simulink library "mcadROM_lib"  (R2021b)
settings: Solver=VariableStepAuto  StartTime=0.0  StopTime=10.0  RelTol=1e-3
undefined symbols (not defined in the file): AdjMat, Banding_Loss_Mat, Friction_Loss_Mat, idx_TcoolantIn, idx_TcoolantOut, Iron_Loss_Rotor_Back_Iron_Mat, Iron_Loss_Rotor_Pole_Mat, Iron_Loss_Rotor_Tooth_Mat, Iron_Loss_Stator_Back_Iron_Mat, Iron_Loss_Stator_Tooth_Mat, Magnet_Loss_Mat, numStates, Rotor_Cage_Loss_Mat, ShaftTorqueVec, Sleeve_Loss_Mat, SpeedVec, StateSpaceND, Stator_Copper_Loss_AC_Mat, Stator_Copper_Loss_Mat, Stray_Load_Loss_Mat, Stray_Loss_Stator_Iron_Proportion, TnodesInit, Windage_Loss_Mat
libraries: cstblocks x2
settings Model: Creator=agonzale  LastModifiedBy=agonzale

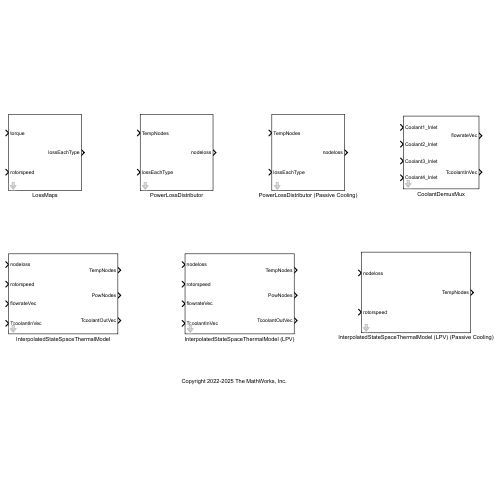
[thumbnail: Simulink's stored preview of the top-level diagram]
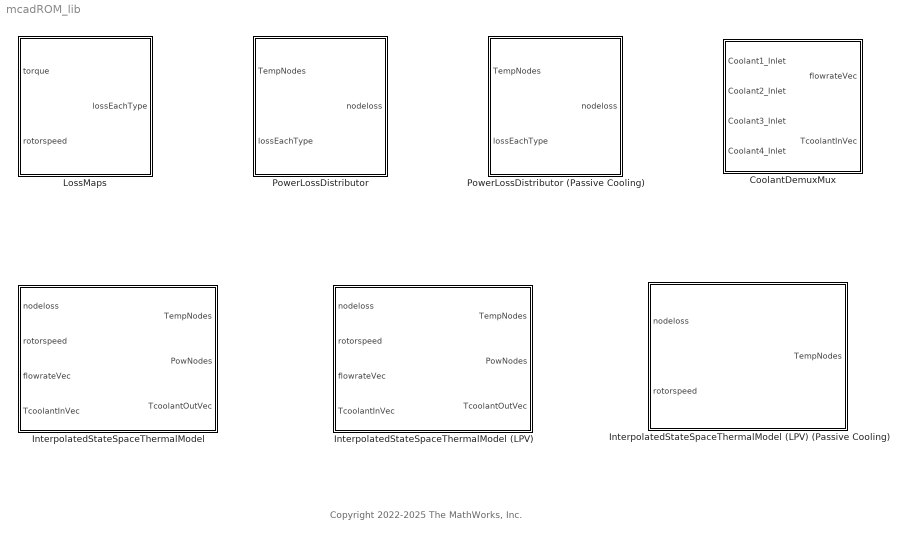
== system mcadROM_lib ==
  note: Copyright 2022-2025 The MathWorks, Inc.
  CoolantDemuxMux : Subsystem  mask{numCoolSys=4}
      mask prompts: numCoolSys "Number of cooling systems"
      mask init:
      | block_in2 = find_system(gcb, ...
      |     'LookUnderMasks', 'on', ...
      |     'FollowLinks', 'on', 'Name', 'Coolant2_Inlet');
      | 
      | block_in3 = find_system(gcb, ...
      |     'LookUnderMasks', 'on', ...
      |     'FollowLinks', 'on', 'Name', 'Coolant3_Inlet');
      | 
      | block_in4 = find_system(gcb, ...
      |     'LookUnderMasks', 'on', ...
      |     'FollowLinks', 'on', 'Name', 'Coolant4_Inlet');
      | 
      | ground2 = find_system(gcb, ...
      |     'LookUnderMasks', 'on', ...
      |     'FollowLinks', 'on', 'Name', 'Ground2');
      | 
      | ground3 = find_system(gcb, ...
      |     'LookUnderMasks', 'on', ...
      |     'FollowLinks', 'on', 'Name', 'Ground3');
      | 
      | ground4 = find_system(gcb, ...
      |     'LookUnderMasks', 'on', ...
      |     'FollowLinks', 'on', 'Name', 'Ground4');
      | 
      | Selector1 = [gcb, '/Selector1'];
      | Selector2 = [gcb, '/Selector2'];
      | 
      | switch numCoolSys
      |     case {1, '1'}
      | 	    set_param(Selector1, 'Indices', '1');
      |         set_param(Selector2, 'Indices', '1');
      |         if ~isempty(block_in2)
      |             delete_line(gcb, 'Coolant2_Inlet/1', 'Demux2/1');
      |             delete_block(block_in2);
      |         end
      |         if ~isempty(block_in3)
      |             delete_line(gcb, 'Coolant3_Inlet/1', 'Demux3/1');
      |             delete_block(block_in3);
      |         end
      |         if ~isempty(block_in4)
      |             delete_line(gcb, 'Coolant4_Inlet/1', 'Demux4/1');
      |             delete_block(block_in4);
      |         end
      |         if isempty(ground2)
      |             add_block('simulink/Sources/Ground', [gcb, '/Ground2']);
      |             add_line(gcb, 'Ground2/1', 'Demux2/1');
      |         end
      |         if isempty(ground3)
      |             add_block('simulink/Sources/Ground', [gcb, '/Ground3']);
      |             add_line(gcb, 'Ground3/1', 'Demux3/1');
      |         end
      |         if isempty(ground4)
      |             add_block('simulink/Sources/Ground', [gcb, '/Ground4']);
      |             add_line(gcb, 'Ground4/1', 'Demux4/1');
      |         end
      |     case {2, '2'}
      |         set_param(Selector1, 'Indices', '[1,2]');
      |         set_param(Selector2, 'Indices', '[1,2]');       
      |         if ~isempty(block_in3)
      |             delete_line(gcb, 'Coolant3_Inlet/1', 'Demux3/1');
      |             delete_block(block_in3);
      |         end
      |         if ~isempty(block_in4)
      |             delete_line(gcb, 'Coolant4_Inlet/1', 'Demux4/1');
      |             delete_block(block_in4);
      |         end 
      |         if ~isempty(ground2)
      |             delete_line(gcb, 'Ground2/1', 'Demux2/1');
      |             delete_block(ground2);
      |         end
      |         if isempty(block_in2)
      |             add_block('built-in/Inport', [gcb, '/Coolant2_Inlet']);
      |             add_line(gcb, 'Coolant2_Inlet/1', 'Demux2/1');
      |         end
      |         if isempty(ground3)
      |             add_block('simulink/Sources/Ground', [gcb, '/Ground3']);
      |             add_line(gcb, 'Ground3/1', 'Demux3/1');
      |         end
      |         if isempty(ground4)
      |             add_block('simulink/Sources/Ground', [gcb, '/Ground4']);
      |             add_line(gcb, 'Ground4/1', 'Demux4/1');
      |         end
      |     case {3, '3'}
      |         set_param(Selector1, 'Indices', '[1,2,3]');
      |         set_param(Selector2, 'Indices', '[1,2,3]');       
      |         if ~isempty(block_in4)          
      |             delete_line(gcb, 'Coolant4_Inlet/1', 'Demux4/1');
      |             delete_block(block_in4);
      |         end 
      |         if ~isempty(ground2)
      |             delete_line(gcb, 'Ground2/1', 'Demux2/1');
      |             delete_block(ground2);
      |         end
      |         if ~isempty(ground3)
      |             delete_line(gcb, 'Ground3/1', 'Demux3/1');
      |             delete_block(ground3);         
      |         end
      |         if isempty(block_in2)
      |             add_block('built-in/Inport', [gcb, '/Coolant2_Inlet']);
      |             add_line(gcb, 'Coolant2_Inlet/1', 'Demux2/1');
      |         end
      |         if isempty(block_in3)
      |             add_block('built-in/Inport', [gcb, '/Coolant3_Inlet']);
      |             add_line(gcb, 'Coolant3_Inlet/1', 'Demux3/1');
      |         end
      |         if isempty(ground4)
      |             add_block('simulink/Sources/Ground', [gcb, '/Ground4']);
      |             add_line(gcb, 'Ground4/1', 'Demux4/1');
      |         end
      |     case {4, '4'}
      |         set_param(Selector1, 'Indices', '[1,2,3,4]');
      |         set_param(Selector2, 'Indices', '[1,2,3,4]');
      |         if ~isempty(ground2)
      |             delete_line(gcb, 'Ground2/1', 'Demux2/1');
      |             delete_block(ground2);
      |         end
      |         if ~isempty(ground3)
      |             delete_line(gcb, 'Ground3/1', 'Demux3/1');
      |             delete_block(ground3);         
      |         end
      |         if ~isempty(ground4)
      |             delete_line(gcb, 'Ground4/1', 'Demux4/1');
      |             delete_block(ground4);
      |         end
      |         if isempty(block_in2)
      |             add_block('built-in/Inport', [gcb, '/Coolant2_Inlet']);
      |             add_line(gcb, 'Coolant2_Inlet/1', 'Demux2/1');
      |         end
      |         if isempty(block_in3)
      |             add_block('built-in/Inport', [gcb, '/Coolant3_Inlet']);
      |             add_line(gcb, 'Coolant3_Inlet/1', 'Demux3/1');
      |         end
      |         if isempty(block_in4)
      |             add_block('built-in/Inport', [gcb, '/Coolant4_Inlet']);
      |             add_line(gcb, 'Coolant4_Inlet/1', 'Demux4/1');
      |         end      
      | end
      mask TypeOptions numCoolSys: 1 | 2 | 3 | 4
  InterpolatedStateSpaceThermalModel : Subsystem  mask{BkptsStruct=struct('w', [1000,6000], 'fr1', [1,10], 'Tin1', [20,60]), AMatND=ones(3,2,2,50,50) % dummy value, BMatND=ones(3,2,2,50,50) % dummy value, ResMatND=ones(3,2,2,50,50) % dummy value, CoolAdjMat=zeros(50) % dummy value, CoolantArrayIdxs=[5 25] % dummy value, InletCoolantIdxs=[5] % dummy value, OutletCoolantIdxs=[25] % dummy value, TnodesInit=25*ones(50,1)}
      mask prompts: BkptsStruct "Speed and cooling inlet breakpoints (struct)"; AMatND "State-space A-matrix for each breakpoint"; BMatND "State-space B-matrix for each breakpoint"; ResMatND "Thermal resistance matrix for each breakpoint"; CoolAdjMat "Global cooling digraph adjacency matrix"; CoolantArrayIdxs "Coolant nodes indexes"; InletCoolantIdxs "Inlet node indexes for cooling systems"; OutletCoolantIdxs "Outlet node indexes for cooling systems"; TnodesInit "Initial node temperatures [degC]"
      mask init:
      | numStates = length(TnodesInit);
      | 
      | % numCoolSys = (length(Xcell)-1)/2;
      | % fieldnames = strings(1+2*numCoolSys,1);
      | % fieldNames(1) = "w";
      | % currentIdx = 2;
      | % for idxCool = 1:numCoolSys
      | %     fieldNames(currentIdx) = string(['fr',num2str(idxCool)]);
      | %     currentIdx = currentIdx+1;
      | % end
      | % for idxCool = 1:numCoolSys
      | %     fieldNames(currentIdx) = string(['Tin',num2str(idxCool)]);
      | %     currentIdx = currentIdx+1;
      | % end 
      | % 
      | % Xstruct = cell2struct(Xcell, fieldNames);
      | 
      | % numCoolSys = length(CoolingDataStruct.EnabledCoolingSystemNames);
      | % Xcell = cell(1+2*numCoolSys,1);
      | % Xcell{1} = RotorSpeedBkpts(:)';
      | % currentIdx = 2;
      | % for idxCool = 1:numCoolSys
      | %     Xcell{currentIdx} = CoolingDataStruct.FlowRateBkpts_lpm{idxCool}(:)';
      | %     currentIdx = currentIdx+1;
      | % end
      | % for idxCool = 1:numCoolSys
      | %     Xcell{currentIdx} = CoolingDataStruct.InletTempBkpts_degC{idxCool}(:)';
      | %     currentIdx = currentIdx+1;
      | % end
  InterpolatedStateSpaceThermalModel (LPV) : Subsystem  mask{StateSpaceND=StateSpaceND, CoolAdjMat=AdjMat, CoolantArrayIdxs=[idx_TcoolantIn, idx_TcoolantOut], InletCoolantIdxs=idx_TcoolantIn, OutletCoolantIdxs=idx_TcoolantOut, TnodesInit=TnodesInit}
      mask prompts: StateSpaceND "Array of state-space models"; CoolAdjMat "Global cooling digraph adjacency matrix"; CoolantArrayIdxs "Coolant nodes indexes"; InletCoolantIdxs "Inlet node indexes for cooling systems"; OutletCoolantIdxs "Outlet node indexes for cooling systems"; TnodesInit "Initial node temperatures [degC]"
      mask init:
      | numStates = length(TnodesInit);
  InterpolatedStateSpaceThermalModel (LPV) (Passive Cooling) : Subsystem  mask{StateSpaceND=StateSpaceND, TnodesInit=TnodesInit}
      mask prompts: StateSpaceND "Array of state-space models"; TnodesInit "Initial node temperatures [degC]"
      mask init:
      | numStates = length(TnodesInit);
  LossMaps : Subsystem  mask{ShaftTorqueVec=ShaftTorqueVec, SpeedVec=SpeedVec, Stator_Copper_Loss_Mat=Stator_Copper_Loss_Mat, Rotor_Cage_Loss_Mat=Rotor_Cage_Loss_Mat, Iron_Loss_Stator_Back_Iron_Mat=Iron_Loss_Stator_Back_Iron_Mat, Iron_Loss_Stator_Tooth_Mat=Iron_Loss_Stator_Tooth_Mat, Stray_Loss_Stator_Iron_Proportion=Stray_Loss_Stator_Iron_Proportion, Stray_Load_Loss_Mat=Stray_Load_Loss_Mat, Magnet_Loss_Mat=Magnet_Loss_Mat, Iron_Loss_Rotor_Pole_Mat=Iron_Loss_Rotor_Pole_Mat, Iron_Loss_Rotor_Back_Iron_Mat=Iron_Loss_Rotor_Back_Iron_Mat, Iron_Loss_Rotor_Tooth_Mat=Iron_Loss_Rotor_Tooth_Mat, Friction_Loss_Mat=Friction_Loss_Mat, Windage_Loss_Mat=Windage_Loss_Mat, Stator_Copper_Loss_AC_Mat=Stator_Copper_Loss_AC_Mat, Banding_Loss_Mat=Banding_Loss_Mat, Sleeve_Loss_Mat=Sleeve_Loss_Mat}
      mask prompts: ShaftTorqueVec "Shaft torque vector"; SpeedVec "Shaft speed vector"; Stator_Copper_Loss_Mat "Stator_Copper_Loss matrix"; Rotor_Cage_Loss_Mat "Rotor_Cage_Loss matrix"; Iron_Loss_Stator_Back_Iron_Mat "Iron_Loss_Stator_Back_Iron matrix"; Iron_Loss_Stator_Tooth_Mat "Iron_Loss_Stator_Tooth matrix"; Stray_Loss_Stator_Iron_Proportion "Stray Loss Stator Iron proportion"; Stray_Load_Loss_Mat "Stray_Load_Loss matrix"; Magnet_Loss_Mat "Magnet_Loss matrix"; Iron_Loss_Rotor_Pole_Mat "Iron_Loss_Rotor_Pole matrix"; Iron_Loss_Rotor_Back_Iron_Mat "Iron_Loss_Rotor_Back_Iron matrix"; Iron_Loss_Rotor_Tooth_Mat "Iron_Loss_Rotor_Tooth matrix"; Friction_Loss_Mat "Friction_Loss matrix"; Windage_Loss_Mat "Windage_Loss matrix"; Stator_Copper_Loss_AC_Mat "Stator_Copper_Loss_AC matrix"; Banding_Loss_Mat "Banding_Loss matrix"; Sleeve_Loss_Mat "Sleeve_Loss matrix"
  PowerLossDistributor : Subsystem  mask{TrefStator=20, StatorCopperTempCoefResistivity=1e-5, TrefRotor=20, RotorCopperTempCoefResistivity=1e-5, LossDistrForEachType=zeros(10,50);, CapMat=zeros(50);, CoolantArrayIdxs=[2,3,4]}
      mask prompts: TrefStator "Stator reference temperature [degC]"; StatorCopperTempCoefResistivity "Stator copper resistivity temperature coefficient"; TrefRotor "Rotor reference temperature [degC]"; RotorCopperTempCoefResistivity "Rotor copper resistivity temperature coefficient"; LossDistrForEachType "Node loss distribution for each loss type (array)"; CapMat "Capacitance matrix"; CoolantArrayIdxs "Coolant nodes indexes"
      mask init:
      | [numStates, ~] = size(CapMat);
  PowerLossDistributor (Passive Cooling) : Subsystem  mask{TrefStator=20, StatorCopperTempCoefResistivity=1e-5, TrefRotor=20, RotorCopperTempCoefResistivity=1e-5, LossDistrForEachType=zeros(10,50);, CapMat=zeros(50);}
      mask prompts: TrefStator "Stator reference temperature [degC]"; StatorCopperTempCoefResistivity "Stator copper resistivity temperature coefficient"; TrefRotor "Rotor reference temperature [degC]"; RotorCopperTempCoefResistivity "Rotor copper resistivity temperature coefficient"; LossDistrForEachType "Node loss distribution for each loss type (array)"; CapMat "Capacitance matrix"
      mask init:
      | [numStates, ~] = size(CapMat);

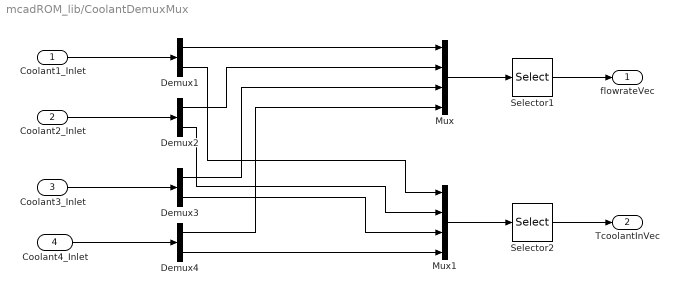
== system mcadROM_lib/CoolantDemuxMux ==
  Coolant1_Inlet : Inport
  Coolant2_Inlet : Inport  Port=2
  Coolant3_Inlet : Inport  Port=3
  Coolant4_Inlet : Inport  Port=4
  Demux{1..4} (4 alike) : Demux  Outputs=2
  Mux : Mux
  Mux1 : Mux
  Selector1 : Selector  InputPortWidth=4  IndexOptions=Index vector (dialog)  Indices=[1,2,3,4]  OutputSizes=1
  Selector2 : Selector  InputPortWidth=4  IndexOptions=Index vector (dialog)  Indices=[1,2,3,4]  OutputSizes=1
  flowrateVec : Outport
  TcoolantInVec : Outport  Port=2
  wires:
  Coolant1_Inlet/1 -> Demux1/1
  Demux1/1 -> Mux/1
  Demux2/1 -> Mux/2
  Demux3/1 -> Mux/3
  Demux4/1 -> Mux/4
  Demux1/2 -> Mux1/1
  Demux2/2 -> Mux1/2
  Demux3/2 -> Mux1/3
  Demux4/2 -> Mux1/4
  Mux/1 -> Selector1/1
  Selector1/1 -> flowrateVec/1
  Mux1/1 -> Selector2/1
  Selector2/1 -> TcoolantInVec/1
  Coolant2_Inlet/1 -> Demux2/1
  Coolant3_Inlet/1 -> Demux3/1
  Coolant4_Inlet/1 -> Demux4/1

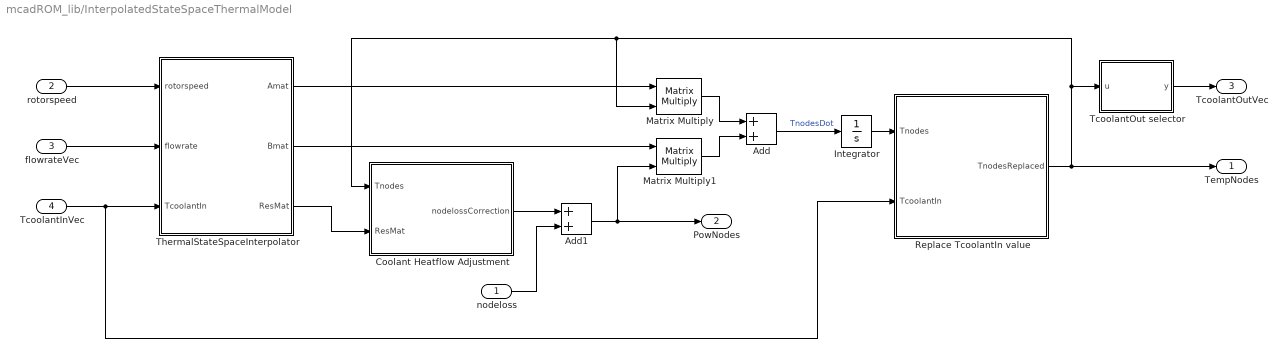
== system mcadROM_lib/InterpolatedStateSpaceThermalModel ==
  nodeloss : Inport
  rotorspeed : Inport  Port=2
  flowrateVec : Inport  Port=3
  TcoolantInVec : Inport  Port=4
  Add : Sum
  Add1 : Sum
  Coolant Heatflow Adjustment : MATLAB Function  TreatAsAtomicUnit=on
  Integrator : Integrator  InitialCondition=TnodesInit
  Matrix Multiply : Product  Multiplication=Matrix(*)
  Matrix Multiply1 : Product  Multiplication=Matrix(*)
  Replace TcoolantIn value : MATLAB Function  TreatAsAtomicUnit=on
  TcoolantOut selector : MATLAB Function  TreatAsAtomicUnit=on
  ThermalStateSpaceInterpolator : MATLAB Function  TreatAsAtomicUnit=on
  TempNodes : Outport
  PowNodes : Outport  Port=2
  TcoolantOutVec : Outport  Port=3
  wires:
  TcoolantOut selector/1(y) -> TcoolantOutVec/1
  Add1/1 -> PowNodes/1, Matrix Multiply1/2
  Matrix Multiply1/1 -> Add/2
  Integrator/1 -> Replace TcoolantIn value/1(Tnodes)
  Add/1 -> Integrator/1  "TnodesDot"
  Coolant Heatflow Adjustment/1(nodelossCorrection) -> Add1/1
  Matrix Multiply/1 -> Add/1
  Replace TcoolantIn value/1(TnodesReplaced) -> TempNodes/1, TcoolantOut selector/1(u), Matrix Multiply/2, Coolant Heatflow Adjustment/1(Tnodes)
  nodeloss/1 -> Add1/2
  TcoolantInVec/1 -> ThermalStateSpaceInterpolator/3(TcoolantIn), Replace TcoolantIn value/2(TcoolantIn)
  rotorspeed/1 -> ThermalStateSpaceInterpolator/1(rotorspeed)
  flowrateVec/1 -> ThermalStateSpaceInterpolator/2(flowrate)
  ThermalStateSpaceInterpolator/1(Amat) -> Matrix Multiply/1
  ThermalStateSpaceInterpolator/2(Bmat) -> Matrix Multiply1/1
  ThermalStateSpaceInterpolator/3(ResMat) -> Coolant Heatflow Adjustment/2(ResMat)

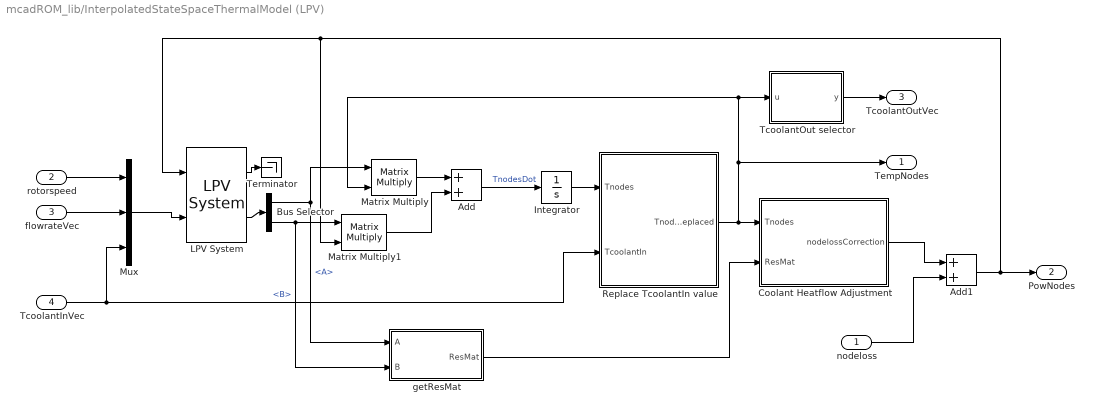
== system mcadROM_lib/InterpolatedStateSpaceThermalModel (LPV) ==
  nodeloss : Inport
  rotorspeed : Inport  Port=2
  flowrateVec : Inport  Port=3
  TcoolantInVec : Inport  Port=4
  Add : Sum
  Add1 : Sum
  Bus Selector : BusSelector  OutputSignals=A,B
  Coolant Heatflow Adjustment : MATLAB Function  TreatAsAtomicUnit=on
  Integrator : Integrator  InitialCondition=TnodesInit
  LPV System : cstblocks/Linear Parameter Varying/LPV System  sys=StateSpaceND  x0=TnodesInit  uOffset=0  yOffset=0  xOffset=0  opEquilOption=on  dxOffset=0  sysFixedOption=Use the first model in state-space array  sysFixed=[]  AFixed=false  BFixed=false  CFixed=false  DFixed=false  uDelayFixed=false  yDelayFixed=false  iDelayFixed=false  IMethod=Linear  EMethod=Clip  IndexSearch=Binary search  IndexBegin=on  OutputX=off  OutputXdot=off  OutputLTI=on  OutputOP=off  DataType=double  SimMode=Interpreted execution  InitBufferSize=1024  FixedBuffer=off
      settings: SourceProductBaseCode=CT
  Matrix Multiply : Product  Multiplication=Matrix(*)
  Matrix Multiply1 : Product  Multiplication=Matrix(*)
  Mux : Mux  Inputs=3
  Replace TcoolantIn value : MATLAB Function  TreatAsAtomicUnit=on
  TcoolantOut selector : MATLAB Function  TreatAsAtomicUnit=on
  Terminator : Terminator
  getResMat : MATLAB Function  TreatAsAtomicUnit=on
  TempNodes : Outport
  PowNodes : Outport  Port=2
  TcoolantOutVec : Outport  Port=3
  wires:
  Bus Selector/1 -> getResMat/1(A), Matrix Multiply/1  "<A>"
  LPV System/2 -> Bus Selector/1
  Integrator/1 -> Replace TcoolantIn value/1(Tnodes)
  Matrix Multiply1/1 -> Add/2
  Replace TcoolantIn value/1(TnodesReplaced) -> TempNodes/1, Matrix Multiply/2, TcoolantOut selector/1(u), Coolant Heatflow Adjustment/1(Tnodes)
  Matrix Multiply/1 -> Add/1
  Add/1 -> Integrator/1  "TnodesDot"
  Add1/1 -> PowNodes/1, LPV System/1, Matrix Multiply1/2
  Bus Selector/2 -> getResMat/2(B), Matrix Multiply1/1  "<B>"
  Coolant Heatflow Adjustment/1(nodelossCorrection) -> Add1/1
  getResMat/1(ResMat) -> Coolant Heatflow Adjustment/2(ResMat)
  Mux/1 -> LPV System/2
  TcoolantInVec/1 -> Replace TcoolantIn value/2(TcoolantIn), Mux/3
  nodeloss/1 -> Add1/2
  flowrateVec/1 -> Mux/2
  rotorspeed/1 -> Mux/1
  TcoolantOut selector/1(y) -> TcoolantOutVec/1
  LPV System/1 -> Terminator/1

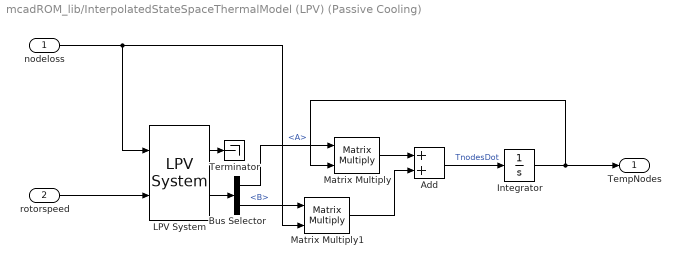
== system mcadROM_lib/InterpolatedStateSpaceThermalModel (LPV) (Passive Cooling) ==
  nodeloss : Inport
  rotorspeed : Inport  Port=2
  Add : Sum
  Bus Selector : BusSelector  OutputSignals=A,B
  Integrator : Integrator  InitialCondition=TnodesInit
  LPV System : cstblocks/Linear Parameter Varying/LPV System  sys=StateSpaceND  x0=TnodesInit  uOffset=0  yOffset=0  xOffset=0  opEquilOption=on  dxOffset=0  sysFixedOption=Use the first model in state-space array  sysFixed=[]  AFixed=false  BFixed=false  CFixed=false  DFixed=false  uDelayFixed=false  yDelayFixed=false  iDelayFixed=false  IMethod=Linear  EMethod=Clip  IndexSearch=Binary search  IndexBegin=on  OutputX=off  OutputXdot=off  OutputLTI=on  OutputOP=off  DataType=double  SimMode=Interpreted execution  InitBufferSize=1024  FixedBuffer=off
      settings: SourceProductBaseCode=CT
  Matrix Multiply : Product  Multiplication=Matrix(*)
  Matrix Multiply1 : Product  Multiplication=Matrix(*)
  Terminator : Terminator
  TempNodes : Outport
  wires:
  Bus Selector/1 -> Matrix Multiply/1  "<A>"
  LPV System/2 -> Bus Selector/1
  Matrix Multiply1/1 -> Add/2
  Integrator/1 -> Matrix Multiply/2, TempNodes/1
  Matrix Multiply/1 -> Add/1
  Add/1 -> Integrator/1  "TnodesDot"
  Bus Selector/2 -> Matrix Multiply1/1  "<B>"
  rotorspeed/1 -> LPV System/2
  LPV System/1 -> Terminator/1
  nodeloss/1 -> Matrix Multiply1/2, LPV System/1

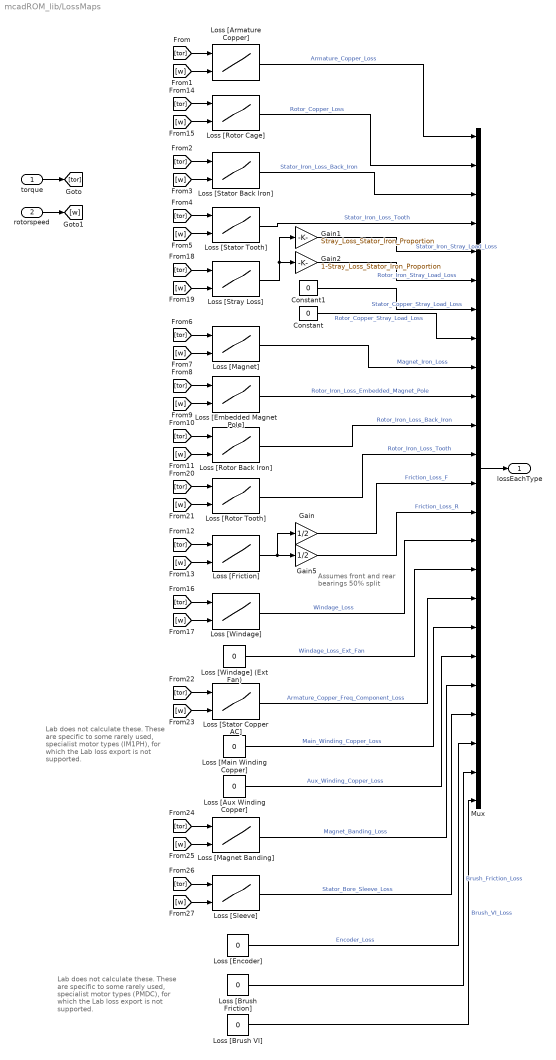
== system mcadROM_lib/LossMaps ==
  note: Lab does not calculate these.
      | These are specific to some rarely used, specialist  motor types (IM1PH), for which the Lab loss export is not supported.
  note: Assumes front and rear bearings 50% split
  note: Lab does not calculate these.
      | These are specific to some rarely used, specialist  motor types (PMDC), for which the Lab loss export is not supported.
  torque : Inport
  rotorspeed : Inport  Port=2
  Constant : Constant  Value=0
  Constant1 : Constant  Value=0
  Gain : Gain  Gain=1/2
  Gain1 : Gain  Gain=Stray_Loss_Stator_Iron_Proportion
  Gain2 : Gain  Gain=1-Stray_Loss_Stator_Iron_Proportion
  Gain5 : Gain  Gain=1/2
  Loss [Armature Copper] : Lookup_n-D  BreakpointsForDimension1=ShaftTorqueVec  BreakpointsForDimension2=SpeedVec  Table=Stator_Copper_Loss_Mat  ExtrapMethod=Clip  UseLastTableValue=on  InternalRulePriority=Speed  RndMeth=Simplest  InputSameDT=on
      settings: InputPortMap=u0,u1
  Loss [Aux Winding Copper] : Constant  Value=0
  Loss [Brush Friction] : Constant  Value=0
  Loss [Brush VI] : Constant  Value=0
  Loss [Embedded Magnet Pole] : Lookup_n-D  BreakpointsForDimension1=ShaftTorqueVec  BreakpointsForDimension2=SpeedVec  Table=Iron_Loss_Rotor_Pole_Mat  ExtrapMethod=Clip  UseLastTableValue=on  InternalRulePriority=Speed  RndMeth=Simplest  InputSameDT=on
      settings: InputPortMap=u0,u1
  Loss [Encoder] : Constant  Value=0
  Loss [Friction] : Lookup_n-D  BreakpointsForDimension1=ShaftTorqueVec  BreakpointsForDimension2=SpeedVec  Table=Friction_Loss_Mat  ExtrapMethod=Clip  UseLastTableValue=on  InternalRulePriority=Speed  RndMeth=Simplest  InputSameDT=on
      settings: InputPortMap=u0,u1
  Loss [Magnet Banding] : Lookup_n-D  BreakpointsForDimension1=ShaftTorqueVec  BreakpointsForDimension2=SpeedVec  Table=Banding_Loss_Mat  ExtrapMethod=Clip  UseLastTableValue=on  InternalRulePriority=Speed  RndMeth=Simplest  InputSameDT=on
      settings: InputPortMap=u0,u1
  Loss [Magnet] : Lookup_n-D  BreakpointsForDimension1=ShaftTorqueVec  BreakpointsForDimension2=SpeedVec  Table=Magnet_Loss_Mat  ExtrapMethod=Clip  UseLastTableValue=on  InternalRulePriority=Speed  RndMeth=Simplest  InputSameDT=on
      settings: InputPortMap=u0,u1
  Loss [Main Winding Copper] : Constant  Value=0
  Loss [Rotor Back Iron] : Lookup_n-D  BreakpointsForDimension1=ShaftTorqueVec  BreakpointsForDimension2=SpeedVec  Table=Iron_Loss_Rotor_Back_Iron_Mat  ExtrapMethod=Clip  UseLastTableValue=on  InternalRulePriority=Speed  RndMeth=Simplest  InputSameDT=on
      settings: InputPortMap=u0,u1
  Loss [Rotor Cage] : Lookup_n-D  BreakpointsForDimension1=ShaftTorqueVec  BreakpointsForDimension2=SpeedVec  Table=Rotor_Cage_Loss_Mat  ExtrapMethod=Clip  UseLastTableValue=on  InternalRulePriority=Speed  RndMeth=Simplest  InputSameDT=on
      settings: InputPortMap=u0,u1
  Loss [Rotor Tooth] : Lookup_n-D  BreakpointsForDimension1=ShaftTorqueVec  BreakpointsForDimension2=SpeedVec  Table=Iron_Loss_Rotor_Tooth_Mat  ExtrapMethod=Clip  UseLastTableValue=on  InternalRulePriority=Speed  RndMeth=Simplest  InputSameDT=on
      settings: InputPortMap=u0,u1
  Loss [Sleeve] : Lookup_n-D  BreakpointsForDimension1=ShaftTorqueVec  BreakpointsForDimension2=SpeedVec  Table=Sleeve_Loss_Mat  ExtrapMethod=Clip  UseLastTableValue=on  InternalRulePriority=Speed  RndMeth=Simplest  InputSameDT=on
      settings: InputPortMap=u0,u1
  Loss [Stator Back Iron] : Lookup_n-D  BreakpointsForDimension1=ShaftTorqueVec  BreakpointsForDimension2=SpeedVec  Table=Iron_Loss_Stator_Back_Iron_Mat  ExtrapMethod=Clip  UseLastTableValue=on  InternalRulePriority=Speed  RndMeth=Simplest  InputSameDT=on
      settings: InputPortMap=u0,u1
  Loss [Stator Copper AC] : Lookup_n-D  BreakpointsForDimension1=ShaftTorqueVec  BreakpointsForDimension2=SpeedVec  Table=Stator_Copper_Loss_AC_Mat  ExtrapMethod=Clip  UseLastTableValue=on  InternalRulePriority=Speed  RndMeth=Simplest  InputSameDT=on
      settings: InputPortMap=u0,u1
  Loss [Stator Tooth] : Lookup_n-D  BreakpointsForDimension1=ShaftTorqueVec  BreakpointsForDimension2=SpeedVec  Table=Iron_Loss_Stator_Tooth_Mat  ExtrapMethod=Clip  UseLastTableValue=on  InternalRulePriority=Speed  RndMeth=Simplest  InputSameDT=on
      settings: InputPortMap=u0,u1
  Loss [Stray Loss] : Lookup_n-D  BreakpointsForDimension1=ShaftTorqueVec  BreakpointsForDimension2=SpeedVec  Table=Stray_Load_Loss_Mat  ExtrapMethod=Clip  UseLastTableValue=on  InternalRulePriority=Speed  RndMeth=Simplest  InputSameDT=on
      settings: InputPortMap=u0,u1
  Loss [Windage] : Lookup_n-D  BreakpointsForDimension1=ShaftTorqueVec  BreakpointsForDimension2=SpeedVec  Table=Windage_Loss_Mat  ExtrapMethod=Clip  UseLastTableValue=on  InternalRulePriority=Speed  RndMeth=Simplest  InputSameDT=on
      settings: InputPortMap=u0,u1
  Loss [Windage] (Ext Fan) : Constant  Value=0
  Mux : Mux  Inputs=24
  lossEachType : Outport
  wires:
  torque/1 -> [tor]
  [tor] -> Loss [Rotor Back Iron]/1
  [tor] -> Loss [Embedded Magnet Pole]/1
  [w] -> Loss [Windage]/2
  [w] -> Loss [Friction]/2
  [tor] -> Loss [Friction]/1
  [tor] -> Loss [Stator Tooth]/1
  Loss [Armature Copper]/1 -> Mux/1  "Armature_Copper_Loss"
  [w] -> Loss [Armature Copper]/2
  [w] -> Loss [Magnet]/2
  [w] -> Loss [Stator Tooth]/2
  [tor] -> Loss [Magnet]/1
  Loss [Friction]/1 -> Gain5/1, Gain/1
  [w] -> Loss [Rotor Back Iron]/2
  [w] -> Loss [Embedded Magnet Pole]/2
  [tor] -> Loss [Stator Back Iron]/1
  [tor] -> Loss [Armature Copper]/1
  rotorspeed/1 -> [w]
  [w] -> Loss [Stator Back Iron]/2
  Mux/1 -> lossEachType/1
  [tor] -> Loss [Windage]/1
  [tor] -> Loss [Rotor Cage]/1
  [w] -> Loss [Rotor Cage]/2
  Loss [Rotor Cage]/1 -> Mux/2  "Rotor_Copper_Loss"
  Loss [Stator Back Iron]/1 -> Mux/3  "Stator_Iron_Loss_Back_Iron"
  Loss [Stator Tooth]/1 -> Mux/4  "Stator_Iron_Loss_Tooth"
  [w] -> Loss [Stray Loss]/2
  [tor] -> Loss [Stray Loss]/1
  Loss [Magnet]/1 -> Mux/9  "Magnet_Iron_Loss"
  Gain1/1 -> Mux/5  "Stator_Iron_Stray_Load_Loss"
  Gain2/1 -> Mux/6  "Rotor_Iron_Stray_Load_Loss"
  Constant1/1 -> Mux/7  "Stator_Copper_Stray_Load_Loss"
  Constant/1 -> Mux/8  "Rotor_Copper_Stray_Load_Loss"
  Loss [Stray Loss]/1 -> Gain1/1, Gain2/1
  Loss [Embedded Magnet Pole]/1 -> Mux/10  "Rotor_Iron_Loss_Embedded_Magnet_Pole"
  Loss [Rotor Back Iron]/1 -> Mux/11  "Rotor_Iron_Loss_Back_Iron"
  [w] -> Loss [Rotor Tooth]/2
  [tor] -> Loss [Rotor Tooth]/1
  Loss [Rotor Tooth]/1 -> Mux/12  "Rotor_Iron_Loss_Tooth"
  Gain/1 -> Mux/13  "Friction_Loss_F"
  Gain5/1 -> Mux/14  "Friction_Loss_R"
  Loss [Windage]/1 -> Mux/15  "Windage_Loss"
  Loss [Windage] (Ext Fan)/1 -> Mux/16  "Windage_Loss_Ext_Fan"
  [tor] -> Loss [Stator Copper AC]/1
  [w] -> Loss [Stator Copper AC]/2
  Loss [Stator Copper AC]/1 -> Mux/17  "Armature_Copper_Freq_Component_Loss"
  Loss [Main Winding Copper]/1 -> Mux/18  "Main_Winding_Copper_Loss"
  Loss [Aux Winding Copper]/1 -> Mux/19  "Aux_Winding_Copper_Loss"
  [tor] -> Loss [Magnet Banding]/1
  Loss [Magnet Banding]/1 -> Mux/20  "Magnet_Banding_Loss"
  [w] -> Loss [Magnet Banding]/2
  [w] -> Loss [Sleeve]/2
  [tor] -> Loss [Sleeve]/1
  Loss [Sleeve]/1 -> Mux/21  "Stator_Bore_Sleeve_Loss"
  Loss [Encoder]/1 -> Mux/22  "Encoder_Loss"
  Loss [Brush Friction]/1 -> Mux/23  "Brush_Friction_Loss"
  Loss [Brush VI]/1 -> Mux/24  "Brush_VI_Loss"

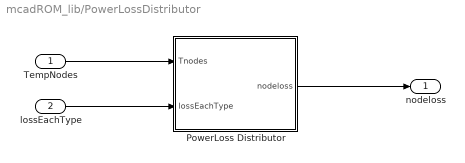
== system mcadROM_lib/PowerLossDistributor ==
  TempNodes : Inport
  lossEachType : Inport  Port=2
  PowerLoss Distributor : MATLAB Function  TreatAsAtomicUnit=on
  nodeloss : Outport
  wires:
  PowerLoss Distributor/1(nodeloss) -> nodeloss/1
  lossEachType/1 -> PowerLoss Distributor/2(lossEachType)
  TempNodes/1 -> PowerLoss Distributor/1(Tnodes)

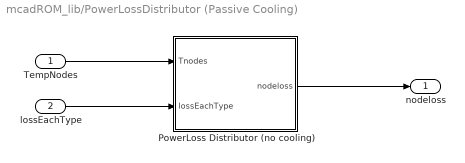
== system mcadROM_lib/PowerLossDistributor (Passive Cooling) ==
  TempNodes : Inport
  lossEachType : Inport  Port=2
  PowerLoss Distributor (no cooling) : MATLAB Function  TreatAsAtomicUnit=on
  nodeloss : Outport
  wires:
  PowerLoss Distributor (no cooling)/1(nodeloss) -> nodeloss/1
  lossEachType/1 -> PowerLoss Distributor (no cooling)/2(lossEachType)
  TempNodes/1 -> PowerLoss Distributor (no cooling)/1(Tnodes)

== matlab function mcadROM_lib/InterpolatedStateSpaceThermalModel (LPV)/getResMat ==
  data: A input; ResMat output; B input
function ResMat = getResMat(A,B)

[ResMat,~] = mcadROM.mfun.getRCFromAB(A,B);

== matlab function mcadROM_lib/PowerLossDistributor (Passive Cooling)/PowerLoss Distributor (no cooling) ==
  data: Tnodes input; lossEachType input; TrefStator parameter size=1; StatorCopperTempCoefResistivity parameter size=1; TrefRotor parameter size=1; RotorCopperTempCoefResistivity parameter size=1; nodeloss output; LossDistrForEachType parameter; numStates parameter size=1; CapMat parameter
function nodeloss = powerLossDistributor(Tnodes, lossEachType, ...
    TrefStator, StatorCopperTempCoefResistivity, TrefRotor, RotorCopperTempCoefResistivity, LossDistrForEachType, numStates, CapMat)


    coder.extrinsic('mcadROM.mfun.powerLossDistributorImplementation');
    nodeloss = zeros(numStates,1);
    CoolantArrayIdxs = [];
    
    nodeloss(:) = mcadROM.mfun.powerLossDistributorImplementation(Tnodes, lossEachType, ...
        TrefStator, StatorCopperTempCoefResistivity, TrefRotor, RotorCopperTempCoefResistivity, LossDistrForEachType, numStates, CapMat, CoolantArrayIdxs);

== matlab function mcadROM_lib/InterpolatedStateSpaceThermalModel/Coolant Heatflow Adjustment ==
  data: Tnodes input; ResMat input; nodelossCorrection output; CoolAdjMat parameter; CoolantArrayIdxs parameter; numStates parameter size=1
function nodelossCorrection = coolantHeatflowAdjustment(Tnodes, ResMat, CoolAdjMat, CoolantArrayIdxs, numStates)


    coder.extrinsic('mcadROM.mfun.coolantHeatflowAdjustmentImplementation');
    nodelossCorrection = zeros(numStates,1);
    
nodelossCorrection(:) = mcadROM.mfun.coolantHeatflowAdjustmentImplementation(Tnodes, ResMat, CoolAdjMat, CoolantArrayIdxs, numStates);

== matlab function mcadROM_lib/InterpolatedStateSpaceThermalModel/Replace TcoolantIn value ==
  data: Tnodes input; TnodesReplaced output; TcoolantIn input; InletCoolantIdxs parameter
function TnodesReplaced = replaceTcoolantInValue(Tnodes, TcoolantIn, InletCoolantIdxs)

    TnodesReplaced = Tnodes;
    TnodesReplaced(InletCoolantIdxs) = TcoolantIn(:);
end

== matlab function mcadROM_lib/InterpolatedStateSpaceThermalModel/ThermalStateSpaceInterpolator ==
  data: rotorspeed input; Amat output; flowrate input; TcoolantIn input; Bmat output; ResMat output; BkptsStruct parameter; BMatND parameter; ResMatND parameter; numStates parameter size=1; AMatND parameter
function [Amat, Bmat, ResMat] = thermalStateSpaceInterpolator(rotorspeed, flowrate, TcoolantIn, ...
                             BkptsStruct, BMatND, ResMatND, numStates, AMatND)


        coder.extrinsic('mcadROM.mfun.thermalStateSpaceInterpolatorImplementation');
        Amat = zeros(numStates, numStates);
        Bmat = zeros(numStates, numStates);
        ResMat = zeros(numStates, numStates);

 [Amat, Bmat, ResMat] = mcadROM.mfun.thermalStateSpaceInterpolatorImplementation(rotorspeed, flowrate, TcoolantIn, ...
                             BkptsStruct, AMatND, BMatND, ResMatND, numStates);

end

== matlab function mcadROM_lib/InterpolatedStateSpaceThermalModel/TcoolantOut selector ==
  data: u input; y output; OutletCoolantIdxs parameter
function y = fcn(u, OutletCoolantIdxs)

y = u(OutletCoolantIdxs);

== matlab function mcadROM_lib/InterpolatedStateSpaceThermalModel (LPV)/Coolant Heatflow Adjustment ==
  data: Tnodes input; ResMat input; nodelossCorrection output; CoolAdjMat parameter; CoolantArrayIdxs parameter; numStates parameter size=1
function nodelossCorrection = coolantHeatflowAdjustment(Tnodes, ResMat, CoolAdjMat, CoolantArrayIdxs, numStates)


    coder.extrinsic('mcadROM.mfun.coolantHeatflowAdjustmentImplementation');
    nodelossCorrection = zeros(numStates,1);
    
nodelossCorrection(:) = mcadROM.mfun.coolantHeatflowAdjustmentImplementation(Tnodes, ResMat, CoolAdjMat, CoolantArrayIdxs, numStates);

== matlab function mcadROM_lib/PowerLossDistributor/PowerLoss Distributor ==
  data: Tnodes input; lossEachType input; TrefStator parameter size=1; StatorCopperTempCoefResistivity parameter size=1; TrefRotor parameter size=1; RotorCopperTempCoefResistivity parameter size=1; nodeloss output; LossDistrForEachType parameter; numStates parameter size=1; CapMat parameter; CoolantArrayIdxs parameter
function nodeloss = powerLossDistributor(Tnodes, lossEachType, ...
    TrefStator, StatorCopperTempCoefResistivity, TrefRotor, RotorCopperTempCoefResistivity, LossDistrForEachType, numStates, CapMat, CoolantArrayIdxs)


    coder.extrinsic('mcadROM.mfun.powerLossDistributorImplementation');
    nodeloss = zeros(numStates,1);
    
    nodeloss(:) = mcadROM.mfun.powerLossDistributorImplementation(Tnodes, lossEachType, ...
        TrefStator, StatorCopperTempCoefResistivity, TrefRotor, RotorCopperTempCoefResistivity, LossDistrForEachType, numStates, CapMat, CoolantArrayIdxs);

== matlab function mcadROM_lib/InterpolatedStateSpaceThermalModel (LPV)/Replace TcoolantIn value ==
  data: Tnodes input; TnodesReplaced output; TcoolantIn input; InletCoolantIdxs parameter
function TnodesReplaced = replaceTcoolantInValue(Tnodes, TcoolantIn, InletCoolantIdxs)
% Overwrite the node temperatures listed in InletCoolantIdxs with the
% corresponding inlet-coolant temperatures.  Unused positions repeat an
% existing index.
%
% Inputs
%   Tnodes            (nNodes × 1)
%   TcoolantIn        (nCoolants × 1)
%   InletCoolantIdxs  (nCoolants × nNozzlesPerCoolant)
%
% Example
%   Tnodes          = ones(26,1);
%   TcoolantIn      = [25; 35; 45]; % three colants
%   InletCoolantIdxs= [2 2; 5 6; 9 10]; % the first coolant has one inlet, the others have two inlets
%   TnodesReplaced  = replaceTcoolantInValue(Tnodes,TcoolantIn,InletCoolantIdxs);

    idx  = InletCoolantIdxs(:);
    vals = repmat(TcoolantIn,1,size(InletCoolantIdxs,2));
    Tnodes(idx) = vals(:);
    TnodesReplaced = Tnodes;
end

== matlab function mcadROM_lib/InterpolatedStateSpaceThermalModel (LPV)/TcoolantOut selector ==
  data: u input; y output; OutletCoolantIdxs parameter
function y = fcn(u, OutletCoolantIdxs)

y = u(OutletCoolantIdxs);
